simulink model "Inestabilidad"  (R2021a)
settings: Solver=VariableStepAuto  StartTime=0.0  StopTime=10.0  RelTol=1e-3
settings Model: Creator=Santiago  LastModifiedBy=Santiago

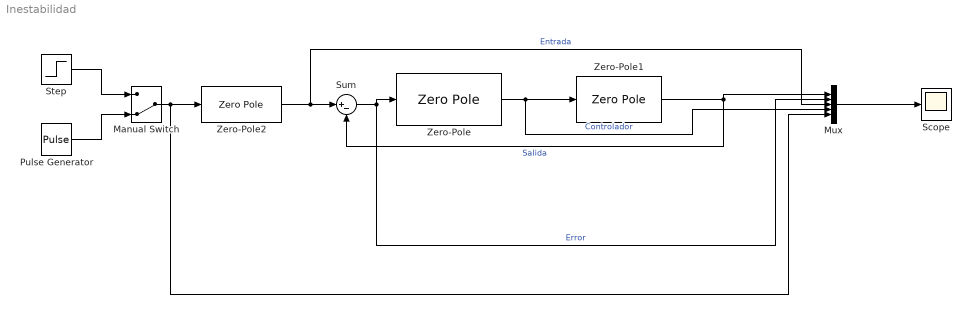
== system Inestabilidad ==
  Manual Switch : ManualSwitch  CurrentSetting=0
  Mux : Mux  Inputs=5
  Pulse Generator : DiscretePulseGenerator  Period=10  PhaseDelay=1
  Scope : Scope
  Step : Step  SampleTime=0
  Sum : Sum  Inputs=|+-
  Zero-Pole : ZeroPole  Zeros=[8 -10]  Poles=[-1 2]
  Zero-Pole1 : ZeroPole  Zeros=[2 -1]  Poles=[0 8]
  Zero-Pole2 : ZeroPole  Zeros=[0]  Poles=[10]
  wires:
  Mux/1 -> Scope/1
  Sum/1 -> Mux/2, Zero-Pole/1  "Error"
  Zero-Pole1/1 -> Sum/2, Mux/1  "Salida"
  Zero-Pole/1 -> Mux/4, Zero-Pole1/1  "Controlador"
  Zero-Pole2/1 -> Mux/3, Sum/1  "Entrada"
  Manual Switch/1 -> Mux/5, Zero-Pole2/1
  Step/1 -> Manual Switch/1
  Pulse Generator/1 -> Manual Switch/2
